simulink model "cruise_control"  (R2025a)
settings: Solver=VariableStepAuto  StartTime=0.0  StopTime=200  RelTol=1e-3
model workspace (MAT data in the model file):
  k1 = Simulink.Parameter
  k1.Value = 2
  k1.Complexity = 'real'
  k1.Dimensions = [1 1]
  k1.DataType = 'auto'
  k2 = Simulink.Parameter
  k2.Value = 100
  k2.Complexity = 'real'
  k2.Dimensions = [1 1]
  k2.DataType = 'auto'
  m = Simulink.Parameter
  m.Value = 1000
  m.Complexity = 'real'
  m.Dimensions = [1 1]
  m.DataType = 'auto'
values from neighbouring files (symbols this model uses):
  k2 = 100    [variable_initialization.m]
  m = 1000    [variable_initialization.m]
libraries: slpidlib x1, SignalEditorBlockLib x1
settings Model: Creator=Potato  LastModifiedBy=Potato

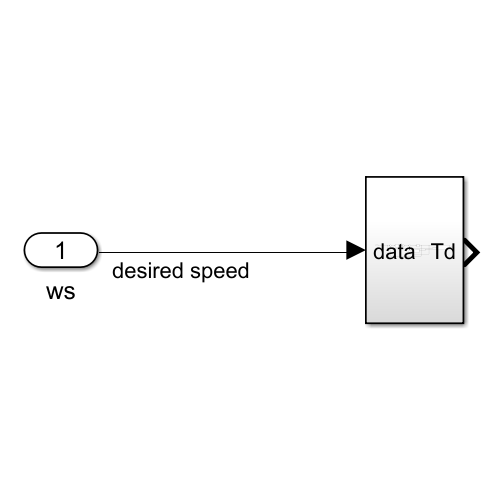
[thumbnail: Simulink's stored preview of the top-level diagram]
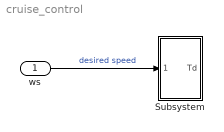
== system cruise_control ==
  ws : Inport
  Subsystem : Subsystem
  wires:
  ws/1 -> Subsystem/1(data)  "desired speed"

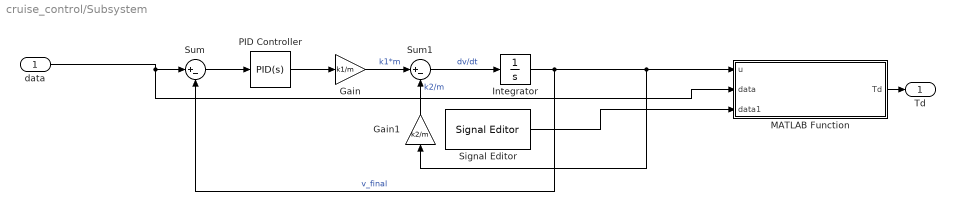
== system cruise_control/Subsystem ==
  data : Inport
  Gain : Gain  Gain=k1/m
  Gain1 : Gain  Gain=k2/m
  Integrator : Integrator  InitialCondition=10
  MATLAB Function : MATLAB Function  TreatAsAtomicUnit=on
  PID Controller : slpidlib/PID Controller  Controller=PID  Form=Parallel  TimeDomain=Continuous-time  UseExternalTs=off  SampleTime=-1  IntegratorMethod=Forward Euler  FilterMethod=Forward Euler  ControllerParametersSource=internal  P=1  I=1  UseKiTs=off  D=0  UseExternalDerivativeSource=off  N=100  UseFilter=on  TunerSelectOption=Transfer Function Based (PID Tuner App)  InitialConditionSource=internal  InitialConditionForIntegrator=0  InitialConditionForFilter=0  DifferentiatorICPrevScaledInput=0  ExternalReset=none  TrackingMode=off  Kt=1  LimitOutput=off  SatLimitsSource=internal  UpperSaturationLimit=inf  LowerSaturationLimit=-inf  LinearizeAsGain=on  AntiWindupMode=none  Kb=1  LimitIntegrator=off  UpperIntegratorSaturationLimit=inf  LowerIntegratorSaturationLimit=-inf  POutMin=[]  POutMax=[]  IOutMin=[]  IOutMax=[]  DOutMin=[]  DOutMax=[]  NOutMin=[]  NOutMax=[]  SumOutMin=[]  SumOutMax=[]  SaturationOutMin=[]  SaturationOutMax=[]  PParamMin=[]  PParamMax=[]  IParamMin=[]  IParamMax=[]  DParamMin=[]  DParamMax=[]  NParamMin=[]  NParamMax=[]  KbParamMin=[]  KbParamMax=[]  KtParamMin=[]  KtParamMax=[]  KbOutMin=[]  KbOutMax=[]  KtOutMin=[]  KtOutMax=[]  IntegratorOutMin=[]  IntegratorOutMax=[]  FilterOutMin=[]  FilterOutMax=[]  SumI1OutMin=[]  SumI1OutMax=[]  SumI2OutMin=[]  SumI2OutMax=[]  SumI3OutMin=[]  SumI3OutMax=[]  SumI4OutMin=[]  SumI4OutMax=[]  SumDOutMin=[]  SumDOutMax=[]  DifferentiatorOutMin=[]  DifferentiatorOutMax=[]  FilterDiffOutCoefMin=[]  FilterDiffOutCoefMax=[]  ReciprocalOutMin=[]  ReciprocalOutMax=[]  SumDenOutMin=[]  SumDenOutMax=[]  SumNumOutMin=[]  SumNumOutMax=[]  DivideOutMin=[]  DivideOutMax=[]  UdiffTsProdOutMin=[]  UdiffTsProdOutMax=[]  NTsProdOutMin=[]  NTsProdOutMax=[]  UintegralTsProdOutMin=[]  UintegralTsProdOutMax=[]  UngainTsProdOutMin=[]  UngainTsProdOutMax=[]  ClampingZeroOutDataTypeStr=Inherit: Inherit via back propagation  ClampingZeroOutMin=[]  ClampingZeroOutMax=[]  FilterDenConstantOutDataTypeStr=Inherit: Inherit via back propagation  FilterDenConstantOutMin=[]  FilterDenConstantOutMax=[]  PCopyOutDataTypeStr=Inherit: Inherit via back propagation  PCopyOutMin=[]  PCopyOutMax=[]  NCopyOutDataTypeStr=Inherit: Inherit via back propagation  NCopyOutMin=[]  NCopyOutMax=[]  IntegratorContinuousStateAttributes=''  IntegratorStateMustResolveToSignalObject=off  IntegratorRTWStateStorageClass=Auto  FilterContinuousStateAttributes=''  FilterStateMustResolveToSignalObject=off  FilterRTWStateStorageClass=Auto  ParallelPVariant=InternalParameters  IdealPVariant=Disabled  IVariant=InternalParameters  DVariant=InternalParameters  IntegratorVariant=Continuous  SatVariant=Disabled  AWVariant=Passthrough  PCopyVariant=Disabled  TRVariant=Disabled  FdbkBlocksVariant=Forward  IdealPFdbkVariant=Disabled  SatFdbkVariant=Disabled  DerivativeFilterVariant=ContFilter  NVariant=InternalParameters  NCopyVariant=Disabled  FilterICVariant=InternalICsFilter  IntegratorICVariant=InternalICs  ExternalResetVariant=Disabled  TRSumVariant=Passthrough  SumFdbkVariant=Disabled  SumVariant=Sum_PID  TsampFilterVariant=InternalTs  TsampNgainVariant=Passthrough  TsampIntegralVariant=Disabled_SignalSpec  ExternalSaturationOutDataTypeStr=Inherit: Same as second input  DerivativeSourceVariant=ErrorSignal  PreIntVariant=InternalPreInt
  Signal Editor : SignalEditorBlockLib/Signal Editor  FileName=C:\Users\Potato\Desktop\EV-Controller\simulink\models\testsig1.mat  ActiveScenario=Scenario  ActiveSignal=Signal 1  IsBus=off  OutputBusObjectStr=Bus: BusObject  SampleTime=0  ZeroCross=off  OutputAfterFinalValue=Setting to zero  Unit=inherit  PreserveSignalName=on  ApplySigPropsToAllScenarios=on  ApplySigPropsToAllSignals=off  SignalPropertySource=Dialog parameters
  Sum : Sum  Inputs=|+-
  Sum1 : Sum  Inputs=|+-
  Td : Outport
  wires:
  Sum1/1 -> Integrator/1  "dv/dt"
  Gain1/1 -> Sum1/2  "k2/m"
  Signal Editor/1 -> MATLAB Function/3(data1)
  Integrator/1 -> MATLAB Function/1(u), Gain1/1, Sum/2  "v_final"
  data/1 -> MATLAB Function/2(data), Sum/1
  Gain/1 -> Sum1/1  "k1*m"
  PID Controller/1 -> Gain/1
  Sum/1 -> PID Controller/1
  MATLAB Function/1(Td) -> Td/1

== matlab function cruise_control/Subsystem/MATLAB Function ==
  data: u input; data input; data1 input; Td output
function Td = velocity_to_torque(u, data, data1)
% u       -> current velocity (v_final from integrator)
% data    -> desired velocity
% data1   -> slope angle in degrees (wave amplitude)

%% 1. Constants
m      = 1000;       % vehicle mass (kg)
rw     = 0.3;        % wheel radius (m)
Ng     = 9;          % gear ratio
eta_dt = 1;          % drivetrain efficiency
k2     = 100;        % linear drag coefficient (N·s/m)
a_f    = 100;        % rolling/friction force (N)
g      = 9.81;       % gravity (m/s^2)
Kp     = 1.0;        % velocity-to-acceleration proportional gain

%% 2. Inputs mapping
v_meas   = u;           % current velocity
v_des    = data;        % desired velocity
slope_deg = data1;      % slope in degrees
A_rad    = slope_deg * pi / 180;  % convert to radians

%% 3. Desired acceleration
err    = v_des - v_meas;
a_des  = Kp * err;

%% 4. Required force at wheels
F_req = m*a_des + k2*v_meas + a_f + m*g*sin(A_rad);

%% 5. Desired torque at motor
Td = (F_req * rw) / (Ng * eta_dt);

end
